simulink model "demapper_simulink"  (R2023a)
settings: Solver=VariableStepAuto  StartTime=0.0  StopTime=976  RelTol=1e-3
libraries: simulink x6
settings Model: Creator=usradmin  LastModifiedBy=usradmin

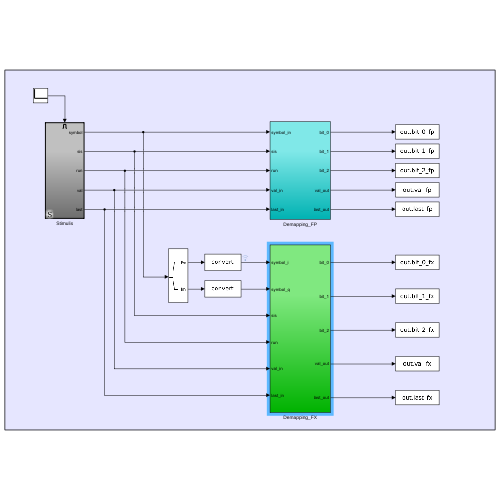
[thumbnail: Simulink's stored preview of the top-level diagram]
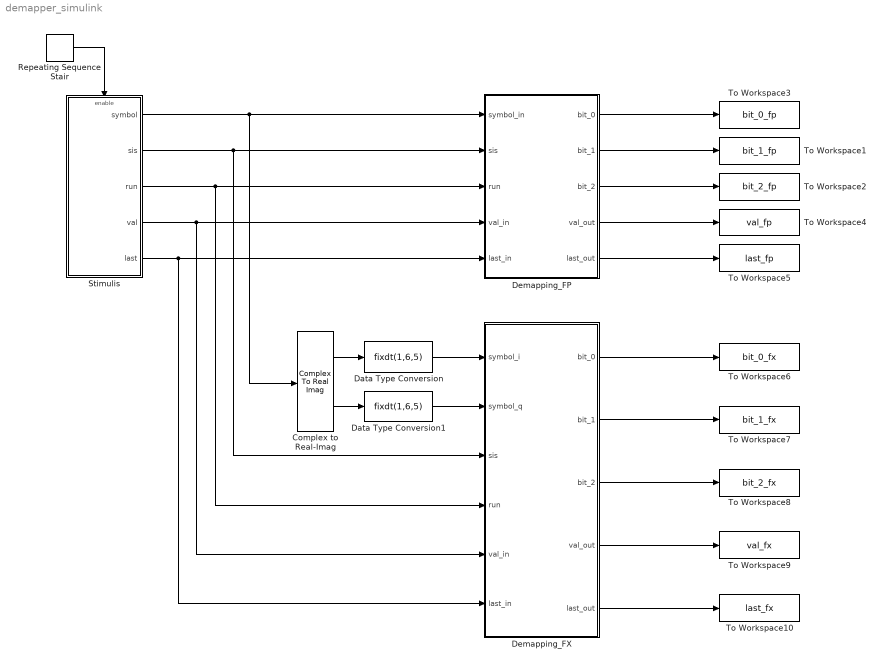
== system demapper_simulink ==
  Complex to Real-Imag : ComplexToRealImag
  Data Type Conversion : DataTypeConversion  OutDataTypeStr=fixdt(1,6,5)  SaturateOnIntegerOverflow=off  RndMeth=Floor
  Data Type Conversion1 : DataTypeConversion  OutDataTypeStr=fixdt(1,6,5)  SaturateOnIntegerOverflow=off  RndMeth=Floor
  Demapping_FP : Subsystem
  Demapping_FX : Subsystem
  Repeating Sequence Stair : simulink/Sources/Repeating Sequence Stair  OutValues=[1].'  tsamp=1  OutMin=[]  OutMax=[]  OutDataTypeStr=double  OutputDataTypeScalingMode=double  OutDataType=fixdt(0,8)  ConRadixGroup=Best Precision: Vector-wise  OutScaling=2^-12
  Stimulis : Subsystem
  To Workspace1 : ToWorkspace  VariableName=bit_1_fp  SaveFormat=Timeseries  SampleTime=-1
  To Workspace10 : ToWorkspace  VariableName=last_fx  SaveFormat=Timeseries  SampleTime=-1
  To Workspace2 : ToWorkspace  VariableName=bit_2_fp  SaveFormat=Timeseries  SampleTime=-1
  To Workspace3 : ToWorkspace  VariableName=bit_0_fp  SaveFormat=Timeseries  SampleTime=-1
  To Workspace4 : ToWorkspace  VariableName=val_fp  SaveFormat=Timeseries  SampleTime=-1
  To Workspace5 : ToWorkspace  VariableName=last_fp  SaveFormat=Timeseries  SampleTime=-1
  To Workspace6 : ToWorkspace  VariableName=bit_0_fx  SaveFormat=Timeseries  SampleTime=-1
  To Workspace7 : ToWorkspace  VariableName=bit_1_fx  SaveFormat=Timeseries  SampleTime=-1
  To Workspace8 : ToWorkspace  VariableName=bit_2_fx  SaveFormat=Timeseries  SampleTime=-1
  To Workspace9 : ToWorkspace  VariableName=val_fx  SaveFormat=Timeseries  SampleTime=-1
  wires:
  Repeating Sequence Stair/1 -> Stimulis/Enable
  Data Type Conversion/1 -> Demapping_FX/1(symbol_i)
  Data Type Conversion1/1 -> Demapping_FX/2(symbol_q)
  Stimulis/2(sis) -> Demapping_FX/3(sis), Demapping_FP/2(sis)
  Complex to Real-Imag/1 -> Data Type Conversion/1
  Complex to Real-Imag/2 -> Data Type Conversion1/1
  Stimulis/1(symbol) -> Complex to Real-Imag/1, Demapping_FP/1(symbol_in)
  Stimulis/3(run) -> Demapping_FX/4(run), Demapping_FP/3(run)
  Stimulis/4(val) -> Demapping_FX/5(val_in), Demapping_FP/4(val_in)
  Stimulis/5(last) -> Demapping_FX/6(last_in), Demapping_FP/5(last_in)
  Demapping_FP/1(bit_0) -> To Workspace3/1
  Demapping_FP/2(bit_1) -> To Workspace1/1
  Demapping_FP/3(bit_2) -> To Workspace2/1
  Demapping_FP/4(val_out) -> To Workspace4/1
  Demapping_FP/5(last_out) -> To Workspace5/1
  Demapping_FX/1(bit_0) -> To Workspace6/1
  Demapping_FX/2(bit_1) -> To Workspace7/1
  Demapping_FX/3(bit_2) -> To Workspace8/1
  Demapping_FX/4(val_out) -> To Workspace9/1
  Demapping_FX/5(last_out) -> To Workspace10/1

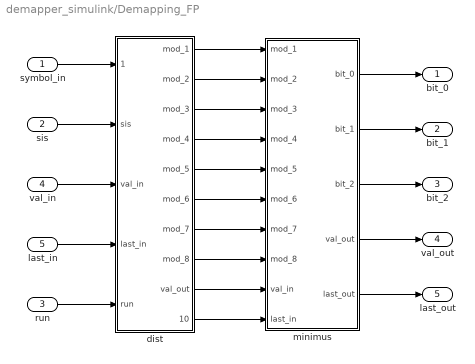
== system demapper_simulink/Demapping_FP ==
  symbol_in : Inport
  sis : Inport  Port=2
  run : Inport  Port=3
  val_in : Inport  Port=4
  last_in : Inport  Port=5
  dist : Subsystem
  minimus : Subsystem
  bit_0 : Outport
  bit_1 : Outport  Port=2
  bit_2 : Outport  Port=3
  val_out : Outport  Port=4
  last_out : Outport  Port=5
  wires:
  minimus/5(last_out) -> last_out/1
  minimus/4(val_out) -> val_out/1
  dist/10(last_out) -> minimus/10(last_in)
  dist/9(val_out) -> minimus/9(val_in)
  run/1 -> dist/5(run)
  last_in/1 -> dist/4(last_in)
  val_in/1 -> dist/3(val_in)
  dist/8(mod_8) -> minimus/8(mod_8)
  dist/7(mod_7) -> minimus/7(mod_7)
  dist/6(mod_6) -> minimus/6(mod_6)
  dist/5(mod_5) -> minimus/5(mod_5)
  dist/4(mod_4) -> minimus/4(mod_4)
  dist/3(mod_3) -> minimus/3(mod_3)
  dist/2(mod_2) -> minimus/2(mod_2)
  minimus/2(bit_1) -> bit_1/1
  minimus/1(bit_0) -> bit_0/1
  dist/1(mod_1) -> minimus/1(mod_1)
  sis/1 -> dist/2(sis)
  minimus/3(bit_2) -> bit_2/1
  symbol_in/1 -> dist/1(symbo_in)

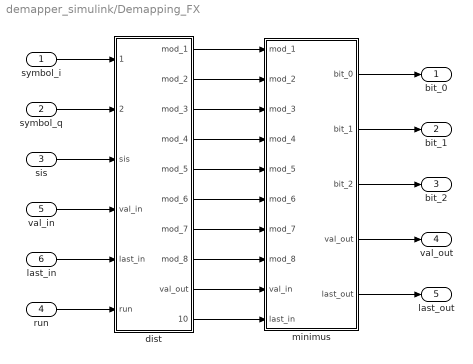
== system demapper_simulink/Demapping_FX ==
  symbol_i : Inport
  symbol_q : Inport  Port=2
  sis : Inport  Port=3
  run : Inport  Port=4
  val_in : Inport  Port=5
  last_in : Inport  Port=6
  dist : Subsystem
  minimus : Subsystem
  bit_0 : Outport
  bit_1 : Outport  Port=2
  bit_2 : Outport  Port=3
  val_out : Outport  Port=4
  last_out : Outport  Port=5
  wires:
  symbol_i/1 -> dist/1(symbol_i)
  symbol_q/1 -> dist/2(symbol_q)
  minimus/3(bit_2) -> bit_2/1
  sis/1 -> dist/3(sis)
  dist/1(mod_1) -> minimus/1(mod_1)
  minimus/1(bit_0) -> bit_0/1
  minimus/2(bit_1) -> bit_1/1
  dist/2(mod_2) -> minimus/2(mod_2)
  dist/3(mod_3) -> minimus/3(mod_3)
  dist/4(mod_4) -> minimus/4(mod_4)
  dist/5(mod_5) -> minimus/5(mod_5)
  dist/6(mod_6) -> minimus/6(mod_6)
  dist/7(mod_7) -> minimus/7(mod_7)
  dist/8(mod_8) -> minimus/8(mod_8)
  val_in/1 -> dist/4(val_in)
  last_in/1 -> dist/5(last_in)
  run/1 -> dist/6(run)
  dist/9(val_out) -> minimus/9(val_in)
  dist/10(last_out) -> minimus/10(last_in)
  minimus/4(val_out) -> val_out/1
  minimus/5(last_out) -> last_out/1

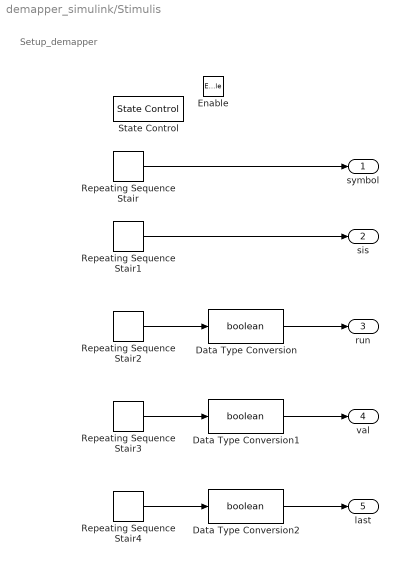
== system demapper_simulink/Stimulis ==
  note: Setup_demapper
  Enable : EnablePort
  Data Type Conversion : DataTypeConversion  OutDataTypeStr=boolean  SaturateOnIntegerOverflow=off  RndMeth=Floor
  Data Type Conversion1 : DataTypeConversion  OutDataTypeStr=boolean  SaturateOnIntegerOverflow=off  RndMeth=Floor
  Data Type Conversion2 : DataTypeConversion  OutDataTypeStr=boolean  SaturateOnIntegerOverflow=off  RndMeth=Floor
  Repeating Sequence Stair : simulink/Sources/Repeating Sequence Stair  OutValues=symbol_cc  tsamp=1  OutMin=[]  OutMax=[]  OutDataTypeStr=double  OutputDataTypeScalingMode=double  OutDataType=fixdt(0,8)  ConRadixGroup=Best Precision: Vector-wise  OutScaling=2^-12
  Repeating Sequence Stair1 : simulink/Sources/Repeating Sequence Stair  OutValues=sis  tsamp=1  OutMin=[]  OutMax=[]  OutDataTypeStr=double  OutputDataTypeScalingMode=double  OutDataType=fixdt(0,8)  ConRadixGroup=Best Precision: Vector-wise  OutScaling=2^-12
  Repeating Sequence Stair2 : simulink/Sources/Repeating Sequence Stair  OutValues=run  tsamp=1  OutMin=[]  OutMax=[]  OutDataTypeStr=double  OutputDataTypeScalingMode=double  OutDataType=fixdt(0,8)  ConRadixGroup=Best Precision: Vector-wise  OutScaling=2^-12
  Repeating Sequence Stair3 : simulink/Sources/Repeating Sequence Stair  OutValues=val  tsamp=1  OutMin=[]  OutMax=[]  OutDataTypeStr=double  OutputDataTypeScalingMode=double  OutDataType=fixdt(0,8)  ConRadixGroup=Best Precision: Vector-wise  OutScaling=2^-12
  Repeating Sequence Stair4 : simulink/Sources/Repeating Sequence Stair  OutValues=last  tsamp=1  OutMin=[]  OutMax=[]  OutDataTypeStr=double  OutputDataTypeScalingMode=double  OutDataType=fixdt(0,8)  ConRadixGroup=Best Precision: Vector-wise  OutScaling=2^-12
  State Control : StateControl  StateControl=Synchronous
  symbol : Outport  VectorParamsAs1DForOutWhenUnconnected=off
  sis : Outport  Port=2  VectorParamsAs1DForOutWhenUnconnected=off
  run : Outport  Port=3  VectorParamsAs1DForOutWhenUnconnected=off
  val : Outport  Port=4  VectorParamsAs1DForOutWhenUnconnected=off
  last : Outport  Port=5  VectorParamsAs1DForOutWhenUnconnected=off
  wires:
  Repeating Sequence Stair/1 -> symbol/1
  Repeating Sequence Stair1/1 -> sis/1
  Repeating Sequence Stair2/1 -> Data Type Conversion/1
  Repeating Sequence Stair3/1 -> Data Type Conversion1/1
  Repeating Sequence Stair4/1 -> Data Type Conversion2/1
  Data Type Conversion/1 -> run/1
  Data Type Conversion1/1 -> val/1
  Data Type Conversion2/1 -> last/1

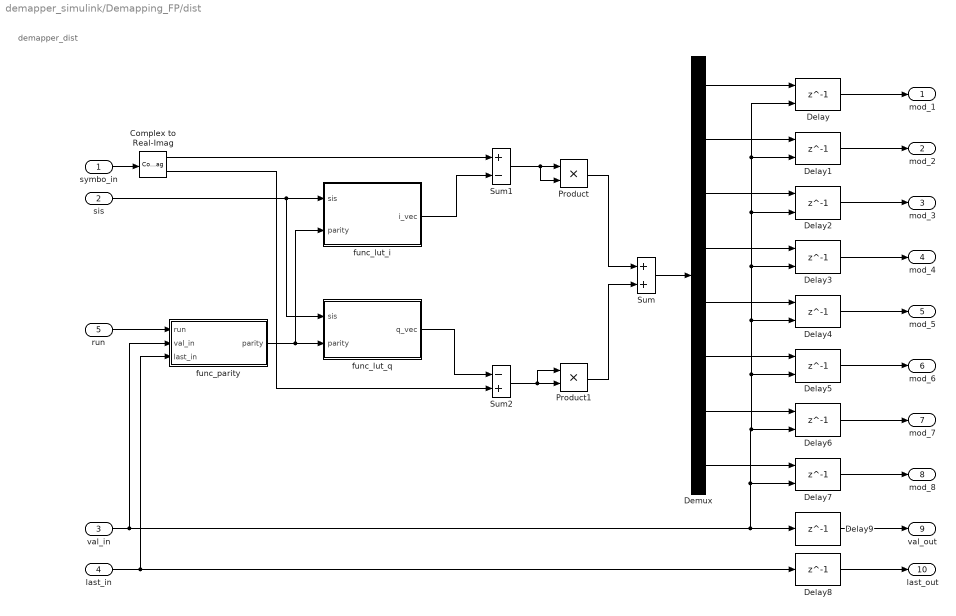
== system demapper_simulink/Demapping_FP/dist ==
  note: demapper_dist
  symbo_in : Inport
  sis : Inport  Port=2
  val_in : Inport  Port=3
  last_in : Inport  Port=4
  run : Inport  Port=5
  Complex to Real-Imag : ComplexToRealImag
  Delay{,1..7} (8 alike) : Delay  DelayLength=1  InitialCondition=0  ShowEnablePort=on
      settings: InputPortMap=u0,e6
  Delay8 : Delay  DelayLength=1  InitialCondition=0
  Delay9 : Delay  DelayLength=1  InitialCondition=0
  Demux : Demux  Outputs=8
  Product : Product
  Product1 : Product
  Sum : Sum
  Sum1 : Sum  Inputs=+-
  Sum2 : Sum  Inputs=-+
  func_lut_i : MATLAB Function  TreatAsAtomicUnit=on
  func_lut_q : MATLAB Function  TreatAsAtomicUnit=on
  func_parity : MATLAB Function  TreatAsAtomicUnit=on
  mod_1 : Outport
  mod_2 : Outport  Port=2
  mod_3 : Outport  Port=3
  mod_4 : Outport  Port=4
  mod_5 : Outport  Port=5
  mod_6 : Outport  Port=6
  mod_7 : Outport  Port=7
  mod_8 : Outport  Port=8
  val_out : Outport  Port=9
  last_out : Outport  Port=10
  wires:
  run/1 -> func_parity/1(run)
  Delay9/1 -> val_out/1
  Delay8/1 -> last_out/1
  last_in/1 -> func_parity/3(last_in), Delay8/1
  Delay7/1 -> mod_8/1
  Delay6/1 -> mod_7/1
  Delay5/1 -> mod_6/1
  Delay4/1 -> mod_5/1
  Delay3/1 -> mod_4/1
  Delay2/1 -> mod_3/1
  Delay1/1 -> mod_2/1
  val_in/1 -> func_parity/2(val_in), Delay9/1, Delay7/2, Delay6/2, Delay5/2, Delay4/2, Delay3/2, Delay2/2, Delay1/2, Delay/2
  Demux/8 -> Delay7/1
  Demux/7 -> Delay6/1
  Demux/6 -> Delay5/1
  Demux/5 -> Delay4/1
  Demux/4 -> Delay3/1
  Demux/3 -> Delay2/1
  Demux/2 -> Delay1/1
  Delay/1 -> mod_1/1
  Demux/1 -> Delay/1
  Sum/1 -> Demux/1
  func_parity/1(parity) -> func_lut_q/2(parity), func_lut_i/2(parity)
  func_lut_q/1(q_vec) -> Sum2/1
  func_lut_i/1(i_vec) -> Sum1/2
  Complex to Real-Imag/2 -> Sum2/2
  Product1/1 -> Sum/2
  Product/1 -> Sum/1
  Sum2/1 -> Product1/2, Product1/1
  sis/1 -> func_lut_i/1(sis), func_lut_q/1(sis)
  Sum1/1 -> Product/1, Product/2
  Complex to Real-Imag/1 -> Sum1/1
  symbo_in/1 -> Complex to Real-Imag/1

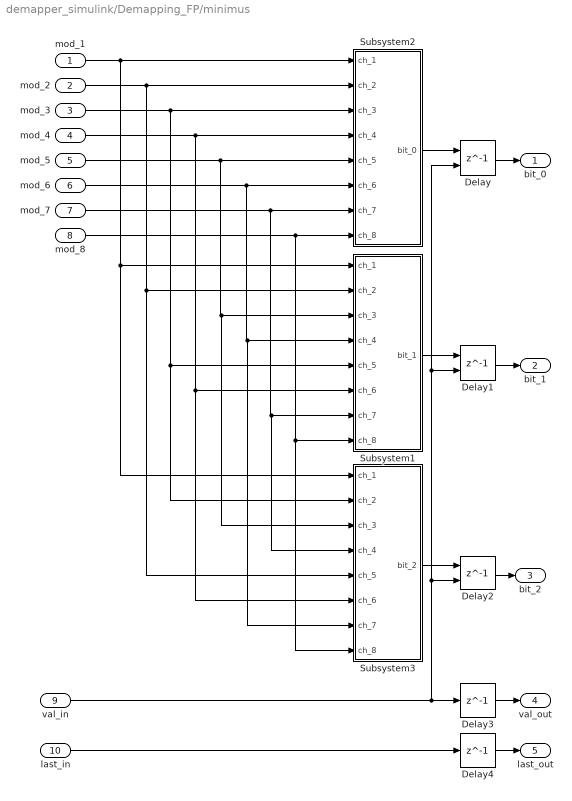
== system demapper_simulink/Demapping_FP/minimus ==
  mod_1 : Inport
  mod_2 : Inport  Port=2
  mod_3 : Inport  Port=3
  mod_4 : Inport  Port=4
  mod_5 : Inport  Port=5
  mod_6 : Inport  Port=6
  mod_7 : Inport  Port=7
  mod_8 : Inport  Port=8
  val_in : Inport  Port=9
  last_in : Inport  Port=10
  Delay : Delay  DelayLength=1  InitialCondition=0  ShowEnablePort=on
      settings: InputPortMap=u0,e6
  Delay1 : Delay  DelayLength=1  InitialCondition=0  ShowEnablePort=on
      settings: InputPortMap=u0,e6
  Delay2 : Delay  DelayLength=1  InitialCondition=0  ShowEnablePort=on
      settings: InputPortMap=u0,e6
  Delay3 : Delay  DelayLength=1  InitialCondition=0
  Delay4 : Delay  DelayLength=1  InitialCondition=0
  Subsystem1 : Subsystem
  Subsystem2 : Subsystem
  Subsystem3 : Subsystem
  bit_0 : Outport  VectorParamsAs1DForOutWhenUnconnected=off
  bit_1 : Outport  Port=2  VectorParamsAs1DForOutWhenUnconnected=off
  bit_2 : Outport  Port=3  VectorParamsAs1DForOutWhenUnconnected=off
  val_out : Outport  Port=4  VectorParamsAs1DForOutWhenUnconnected=off
  last_out : Outport  Port=5  VectorParamsAs1DForOutWhenUnconnected=off
  wires:
  Delay4/1 -> last_out/1
  last_in/1 -> Delay4/1
  Delay3/1 -> val_out/1
  val_in/1 -> Delay3/1, Delay2/2, Delay1/2, Delay/2
  Delay2/1 -> bit_2/1
  Delay1/1 -> bit_1/1
  Delay/1 -> bit_0/1
  mod_7/1 -> Subsystem1/7(ch_7), Subsystem3/4(ch_4), Subsystem2/7(ch_7)
  mod_2/1 -> Subsystem2/2(ch_2), Subsystem1/2(ch_2), Subsystem3/5(ch_5)
  mod_6/1 -> Subsystem3/7(ch_7), Subsystem1/4(ch_4), Subsystem2/6(ch_6)
  mod_1/1 -> Subsystem2/1(ch_1), Subsystem1/1(ch_1), Subsystem3/1(ch_1)
  mod_4/1 -> Subsystem1/6(ch_6), Subsystem3/6(ch_6), Subsystem2/4(ch_4)
  mod_8/1 -> Subsystem3/8(ch_8), Subsystem1/8(ch_8), Subsystem2/8(ch_8)
  Subsystem2/1(bit_0) -> Delay/1
  Subsystem3/1(bit_2) -> Delay2/1
  Subsystem1/1(bit_1) -> Delay1/1
  mod_3/1 -> Subsystem2/3(ch_3), Subsystem3/2(ch_2), Subsystem1/5(ch_5)
  mod_5/1 -> Subsystem2/5(ch_5), Subsystem1/3(ch_3), Subsystem3/3(ch_3)

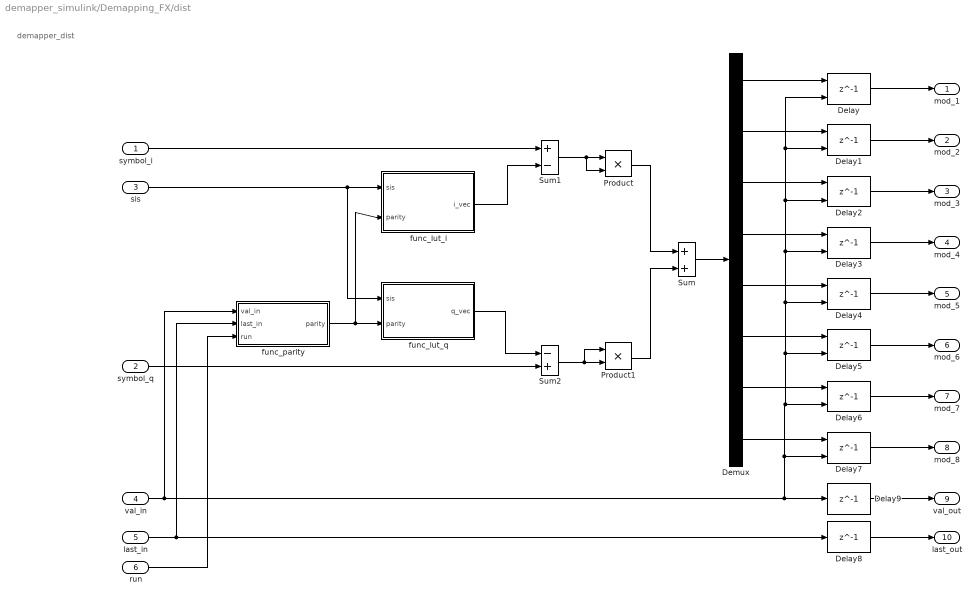
== system demapper_simulink/Demapping_FX/dist ==
  note: demapper_dist
  symbol_i : Inport
  symbol_q : Inport  Port=2
  sis : Inport  Port=3
  val_in : Inport  Port=4
  last_in : Inport  Port=5
  run : Inport  Port=6
  Delay{,1..7} (8 alike) : Delay  DelayLength=1  InitialCondition=0  ShowEnablePort=on
      settings: InputPortMap=u0,e6
  Delay8 : Delay  DelayLength=1  InitialCondition=0
  Delay9 : Delay  DelayLength=1  InitialCondition=0
  Demux : Demux  Outputs=8
  Product : Product
  Product1 : Product
  Sum : Sum
  Sum1 : Sum  Inputs=+-
  Sum2 : Sum  Inputs=-+
  func_lut_i : MATLAB Function  TreatAsAtomicUnit=on
  func_lut_q : MATLAB Function  TreatAsAtomicUnit=on
  func_parity : MATLAB Function  TreatAsAtomicUnit=on
  mod_1 : Outport
  mod_2 : Outport  Port=2
  mod_3 : Outport  Port=3
  mod_4 : Outport  Port=4
  mod_5 : Outport  Port=5
  mod_6 : Outport  Port=6
  mod_7 : Outport  Port=7
  mod_8 : Outport  Port=8
  val_out : Outport  Port=9
  last_out : Outport  Port=10
  wires:
  Sum1/1 -> Product/2, Product/1
  sis/1 -> func_lut_q/1(sis), func_lut_i/1(sis)
  Sum2/1 -> Product1/1, Product1/2
  symbol_i/1 -> Sum1/1
  Product/1 -> Sum/1
  Product1/1 -> Sum/2
  symbol_q/1 -> Sum2/2
  func_lut_i/1(i_vec) -> Sum1/2
  func_lut_q/1(q_vec) -> Sum2/1
  func_parity/1(parity) -> func_lut_i/2(parity), func_lut_q/2(parity)
  Sum/1 -> Demux/1
  Demux/1 -> Delay/1
  Delay/1 -> mod_1/1
  Demux/2 -> Delay1/1
  Demux/3 -> Delay2/1
  Demux/4 -> Delay3/1
  Demux/5 -> Delay4/1
  Demux/6 -> Delay5/1
  Demux/7 -> Delay6/1
  Demux/8 -> Delay7/1
  val_in/1 -> Delay/2, Delay1/2, Delay2/2, Delay3/2, Delay4/2, Delay5/2, Delay6/2, Delay7/2, Delay9/1, func_parity/1(val_in)
  Delay1/1 -> mod_2/1
  Delay2/1 -> mod_3/1
  Delay3/1 -> mod_4/1
  Delay4/1 -> mod_5/1
  Delay5/1 -> mod_6/1
  Delay6/1 -> mod_7/1
  Delay7/1 -> mod_8/1
  last_in/1 -> Delay8/1, func_parity/2(last_in)
  Delay8/1 -> last_out/1
  Delay9/1 -> val_out/1
  run/1 -> func_parity/3(run)

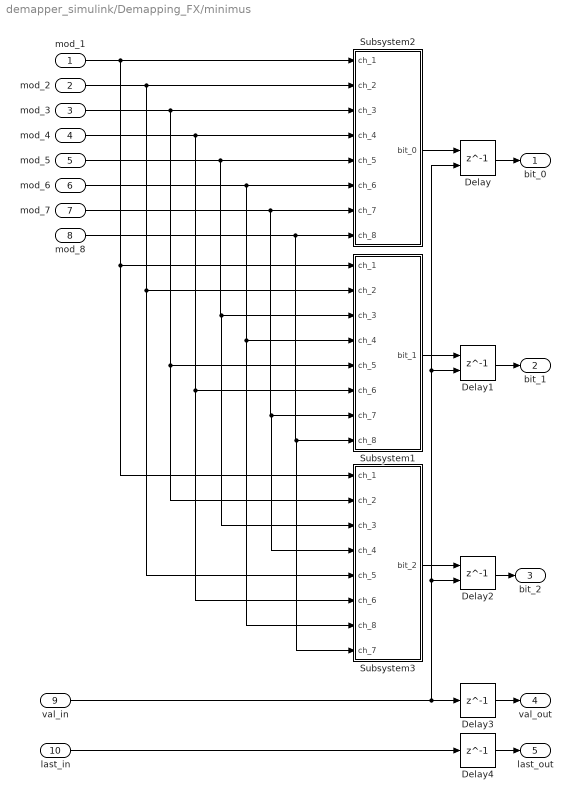
== system demapper_simulink/Demapping_FX/minimus ==
  mod_1 : Inport
  mod_2 : Inport  Port=2
  mod_3 : Inport  Port=3
  mod_4 : Inport  Port=4
  mod_5 : Inport  Port=5
  mod_6 : Inport  Port=6
  mod_7 : Inport  Port=7
  mod_8 : Inport  Port=8
  val_in : Inport  Port=9
  last_in : Inport  Port=10
  Delay : Delay  DelayLength=1  InitialCondition=0  ShowEnablePort=on
      settings: InputPortMap=u0,e6
  Delay1 : Delay  DelayLength=1  InitialCondition=0  ShowEnablePort=on
      settings: InputPortMap=u0,e6
  Delay2 : Delay  DelayLength=1  InitialCondition=0  ShowEnablePort=on
      settings: InputPortMap=u0,e6
  Delay3 : Delay  DelayLength=1  InitialCondition=0
  Delay4 : Delay  DelayLength=1  InitialCondition=0
  Subsystem1 : Subsystem
  Subsystem2 : Subsystem
  Subsystem3 : Subsystem
  bit_0 : Outport  VectorParamsAs1DForOutWhenUnconnected=off
  bit_1 : Outport  Port=2  VectorParamsAs1DForOutWhenUnconnected=off
  bit_2 : Outport  Port=3  VectorParamsAs1DForOutWhenUnconnected=off
  val_out : Outport  Port=4  VectorParamsAs1DForOutWhenUnconnected=off
  last_out : Outport  Port=5  VectorParamsAs1DForOutWhenUnconnected=off
  wires:
  mod_5/1 -> Subsystem3/3(ch_3), Subsystem1/3(ch_3), Subsystem2/5(ch_5)
  mod_3/1 -> Subsystem1/5(ch_5), Subsystem3/2(ch_2), Subsystem2/3(ch_3)
  Subsystem1/1(bit_1) -> Delay1/1
  Subsystem3/1(bit_2) -> Delay2/1
  Subsystem2/1(bit_0) -> Delay/1
  mod_8/1 -> Subsystem2/8(ch_8), Subsystem3/8(ch_7), Subsystem1/8(ch_8)
  mod_4/1 -> Subsystem2/4(ch_4), Subsystem3/6(ch_6), Subsystem1/6(ch_6)
  mod_1/1 -> Subsystem3/1(ch_1), Subsystem1/1(ch_1), Subsystem2/1(ch_1)
  mod_6/1 -> Subsystem2/6(ch_6), Subsystem3/7(ch_8), Subsystem1/4(ch_4)
  mod_2/1 -> Subsystem3/5(ch_5), Subsystem1/2(ch_2), Subsystem2/2(ch_2)
  mod_7/1 -> Subsystem2/7(ch_7), Subsystem3/4(ch_4), Subsystem1/7(ch_7)
  Delay/1 -> bit_0/1
  Delay1/1 -> bit_1/1
  Delay2/1 -> bit_2/1
  val_in/1 -> Delay/2, Delay1/2, Delay2/2, Delay3/1
  Delay3/1 -> val_out/1
  last_in/1 -> Delay4/1
  Delay4/1 -> last_out/1

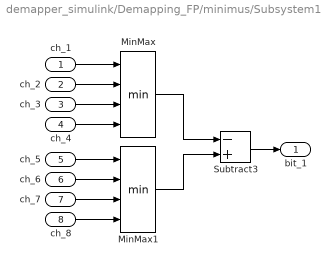
== system demapper_simulink/Demapping_FP/minimus/Subsystem1 ==
  ch_1 : Inport
  ch_2 : Inport  Port=2
  ch_3 : Inport  Port=3
  ch_4 : Inport  Port=4
  ch_5 : Inport  Port=5
  ch_6 : Inport  Port=6
  ch_7 : Inport  Port=7
  ch_8 : Inport  Port=8
  MinMax : MinMax  Inputs=4
  MinMax1 : MinMax  Inputs=4
  Subtract3 : Sum  Inputs=-+
  bit_1 : Outport
  wires:
  ch_7/1 -> MinMax1/3
  ch_8/1 -> MinMax1/4
  Subtract3/1 -> bit_1/1
  ch_5/1 -> MinMax1/1
  MinMax1/1 -> Subtract3/2
  ch_6/1 -> MinMax1/2
  MinMax/1 -> Subtract3/1
  ch_1/1 -> MinMax/1
  ch_3/1 -> MinMax/3
  ch_2/1 -> MinMax/2
  ch_4/1 -> MinMax/4

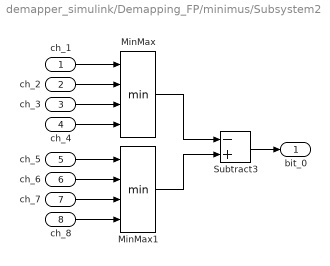
== system demapper_simulink/Demapping_FP/minimus/Subsystem2 ==
  ch_1 : Inport
  ch_2 : Inport  Port=2
  ch_3 : Inport  Port=3
  ch_4 : Inport  Port=4
  ch_5 : Inport  Port=5
  ch_6 : Inport  Port=6
  ch_7 : Inport  Port=7
  ch_8 : Inport  Port=8
  MinMax : MinMax  Inputs=4
  MinMax1 : MinMax  Inputs=4
  Subtract3 : Sum  Inputs=-+
  bit_0 : Outport
  wires:
  ch_4/1 -> MinMax/4
  ch_2/1 -> MinMax/2
  ch_3/1 -> MinMax/3
  ch_1/1 -> MinMax/1
  MinMax/1 -> Subtract3/1
  ch_6/1 -> MinMax1/2
  MinMax1/1 -> Subtract3/2
  ch_5/1 -> MinMax1/1
  Subtract3/1 -> bit_0/1
  ch_8/1 -> MinMax1/4
  ch_7/1 -> MinMax1/3

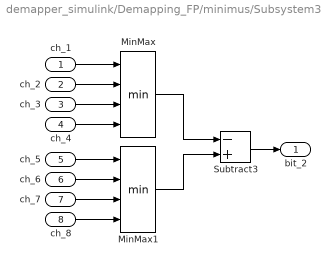
== system demapper_simulink/Demapping_FP/minimus/Subsystem3 ==
  ch_1 : Inport
  ch_2 : Inport  Port=2
  ch_3 : Inport  Port=3
  ch_4 : Inport  Port=4
  ch_5 : Inport  Port=5
  ch_6 : Inport  Port=6
  ch_7 : Inport  Port=7
  ch_8 : Inport  Port=8
  MinMax : MinMax  Inputs=4
  MinMax1 : MinMax  Inputs=4
  Subtract3 : Sum  Inputs=-+
  bit_2 : Outport
  wires:
  ch_4/1 -> MinMax/4
  ch_2/1 -> MinMax/2
  ch_3/1 -> MinMax/3
  ch_1/1 -> MinMax/1
  MinMax/1 -> Subtract3/1
  ch_6/1 -> MinMax1/2
  MinMax1/1 -> Subtract3/2
  ch_5/1 -> MinMax1/1
  Subtract3/1 -> bit_2/1
  ch_8/1 -> MinMax1/4
  ch_7/1 -> MinMax1/3

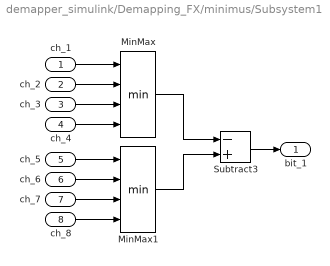
== system demapper_simulink/Demapping_FX/minimus/Subsystem1 ==
  ch_1 : Inport
  ch_2 : Inport  Port=2
  ch_3 : Inport  Port=3
  ch_4 : Inport  Port=4
  ch_5 : Inport  Port=5
  ch_6 : Inport  Port=6
  ch_7 : Inport  Port=7
  ch_8 : Inport  Port=8
  MinMax : MinMax  Inputs=4
  MinMax1 : MinMax  Inputs=4
  Subtract3 : Sum  Inputs=-+
  bit_1 : Outport
  wires:
  ch_4/1 -> MinMax/4
  ch_2/1 -> MinMax/2
  ch_3/1 -> MinMax/3
  ch_1/1 -> MinMax/1
  MinMax/1 -> Subtract3/1
  ch_6/1 -> MinMax1/2
  MinMax1/1 -> Subtract3/2
  ch_5/1 -> MinMax1/1
  Subtract3/1 -> bit_1/1
  ch_8/1 -> MinMax1/4
  ch_7/1 -> MinMax1/3

== system demapper_simulink/Demapping_FX/minimus/Subsystem2 ==
  ch_1 : Inport
  ch_2 : Inport  Port=2
  ch_3 : Inport  Port=3
  ch_4 : Inport  Port=4
  ch_5 : Inport  Port=5
  ch_6 : Inport  Port=6
  ch_7 : Inport  Port=7
  ch_8 : Inport  Port=8
  MinMax : MinMax  Inputs=4
  MinMax1 : MinMax  Inputs=4
  Subtract3 : Sum  Inputs=-+
  bit_0 : Outport
  wires:
  ch_7/1 -> MinMax1/3
  ch_8/1 -> MinMax1/4
  Subtract3/1 -> bit_0/1
  ch_5/1 -> MinMax1/1
  MinMax1/1 -> Subtract3/2
  ch_6/1 -> MinMax1/2
  MinMax/1 -> Subtract3/1
  ch_1/1 -> MinMax/1
  ch_3/1 -> MinMax/3
  ch_2/1 -> MinMax/2
  ch_4/1 -> MinMax/4

== system demapper_simulink/Demapping_FX/minimus/Subsystem3 ==
  ch_1 : Inport
  ch_2 : Inport  Port=2
  ch_3 : Inport  Port=3
  ch_4 : Inport  Port=4
  ch_5 : Inport  Port=5
  ch_6 : Inport  Port=6
  ch_8 : Inport  Port=7
  ch_7 : Inport  Port=8
  MinMax : MinMax  Inputs=4
  MinMax1 : MinMax  Inputs=4
  Subtract3 : Sum  Inputs=-+
  bit_2 : Outport
  wires:
  ch_7/1 -> MinMax1/3
  ch_8/1 -> MinMax1/4
  Subtract3/1 -> bit_2/1
  ch_5/1 -> MinMax1/1
  MinMax1/1 -> Subtract3/2
  ch_6/1 -> MinMax1/2
  MinMax/1 -> Subtract3/1
  ch_1/1 -> MinMax/1
  ch_3/1 -> MinMax/3
  ch_2/1 -> MinMax/2
  ch_4/1 -> MinMax/4

== matlab function demapper_simulink/Demapping_FX/dist/func_lut_q ==
  data: sis input; q_vec output; parity input
function q_vec = func_lut_q(sis, parity)
%#codegen

    if (sis == 1 && parity == 0)
        Q_1 =  0;
        Q_2 =  3;
        Q_3 =  3;
        Q_4 =  3;
        Q_5 =  3;
        Q_6 =  3;
        Q_7 =  0;
        Q_8 =  3;
    
    elseif (sis == 1 && parity == 1)
        Q_1 = 0;
        Q_2 =  3;
        Q_3 =  3;
        Q_4 =  1;
        Q_5 =  3;
        Q_6 = -1;
        Q_7 =  0;
        Q_8 =  3;
    
    elseif (sis == 2 && parity == 0)
        Q_1 =  0; 
        Q_2 =  0.7071;
        Q_3 =  0.7071;
        Q_4 =  1;
        Q_5 = -0.7071;
        Q_6 = -1;
        Q_7 =  0;
        Q_8 = -0.7071;
    
    elseif (sis == 2 && parity == 1)
        Q_1 = 1;
        Q_2 = 3;
        Q_3 = 3;
        Q_4 = 3;
        Q_5 = 3;
        Q_6 = 3;
        Q_7 = -1;
        Q_8 = 3;
    
    elseif (sis == 3 && parity == 0)
        Q_1 =  0.7071; 
        Q_2 =  3;
        Q_3 =  3;
        Q_4 =  0.7071;
        Q_5 =  3;
        Q_6 = -0.7071;
        Q_7 = -0.7071;
        Q_8 =  3;
    
    else
        Q_1 =  0.3827;
        Q_2 =  0.9239;
        Q_3 =  0.3827;
        Q_4 =  0.9239;
        Q_5 = -0.3827;
        Q_6 = -0.9238;
        Q_7 = -0.3827;
        Q_8 = -0.9239;
    end 
    q_vec = [Q_1; Q_2; Q_3; Q_4; Q_5; Q_6; Q_7; Q_8];

end

== matlab function demapper_simulink/Demapping_FX/dist/func_lut_i ==
  data: sis input; i_vec output; parity input
function i_vec = func_lut_i(sis, parity)
%#codegen

    if (sis == 1 && parity == 0)
        I_1 = 1;
        I_2 = 3;
        I_3 = 3;
        I_4 = 3;
        I_5 = 3;
        I_6 = 3;
        I_7 = -1;
        I_8 = 3;
    
    elseif (sis == 1 && parity == 1)
        I_1 = 1;
        I_2 = 3;
        I_3 = 3;
        I_4 = 0;
        I_5 = 3;
        I_6 = 0;
        I_7 = -1;
        I_8 = 3;
    
    elseif (sis == 2 && parity == 0)
        I_1 = 1; 
        I_2 = 0.7071;
        I_3 = -0.7071;
        I_4 = 0;
        I_5 = 0.7071;
        I_6 = 0;
        I_7 = -1;
        I_8 = -0.7071;
    
    elseif (sis == 2 && parity == 1)
        I_1 = 0;
        I_2 = 3;
        I_3 = 3;
        I_4 = 3;
        I_5 = 3;
        I_6 = 3;
        I_7 = 0;
        I_8 = 3;
    
    elseif (sis == 3 && parity == 0)
        I_1 = 0.7071; 
        I_2 = 3;
        I_3 = 3;
        I_4 = -0.7071;
        I_5 = 3;
        I_6 = 0.7071;
        I_7 = -0.7071;
        I_8 = 3;
    
    else
        I_1 = 0.9239;
        I_2 = 0.3827;
        I_3 = -0.9239;
        I_4 = -0.3827;
        I_5 = 0.9239;
        I_6 = 0.3827;
        I_7 = -0.9239;
        I_8 = -0.3827;
    end 
    i_vec = [I_1; I_2; I_3; I_4; I_5; I_6; I_7; I_8];
end

== matlab function demapper_simulink/Demapping_FX/dist/func_parity ==
  data: val_in input; parity output; last_in input; run input
function parity = func_parity(val_in, last_in, run)
% -------------------------------------------------------------------------
% Function valid
% -------------------------------------------------------------------------
    % persistent variable for the state
    persistent count;
    if isempty(count)
        count = uint16(0);
    end

    persistent parity_int;
    if isempty(parity_int)
        parity_int = false;
    end

    % counting up
    if (not(run))
        count = uint16(0);
    elseif (val_in)
        count = count + uint16(1);
        % limit
        if (last_in || count > uint16(156))
            count = uint16(0);
        end
    end

    if (val_in && count > uint16(156))
        parity_int = false;
    elseif (val_in)
        parity_int = not(parity_int);
    end 

    parity = parity_int;
end

== matlab function demapper_simulink/Demapping_FP/dist/func_lut_i ==
  data: sis input; i_vec output; parity input
function i_vec = func_lut_i(sis, parity)
%#codegen

    if (sis == 1 && parity == 0)
        I_1 = 1;
        I_2 = 3;
        I_3 = 3;
        I_4 = 3;
        I_5 = 3;
        I_6 = 3;
        I_7 = -1;
        I_8 = 3;
    
    elseif (sis == 1 && parity == 1)
        I_1 = 1;
        I_2 = 3;
        I_3 = 3;
        I_4 = 0;
        I_5 = 3;
        I_6 = 0;
        I_7 = -1;
        I_8 = 3;
    
    elseif (sis == 2 && parity == 0)
        I_1 = 1; 
        I_2 = 0.7071;
        I_3 = -0.7071;
        I_4 = 0;
        I_5 = 0.7071;
        I_6 = 0;
        I_7 = -1;
        I_8 = -0.7071;
    
    elseif (sis == 2 && parity == 1)
        I_1 = 0;
        I_2 = 3;
        I_3 = 3;
        I_4 = 3;
        I_5 = 3;
        I_6 = 3;
        I_7 = 0;
        I_8 = 3;
    
    elseif (sis == 3 && parity == 0)
        I_1 = 0.7071; 
        I_2 = 3;
        I_3 = 3;
        I_4 = -0.7071;
        I_5 = 3;
        I_6 = 0.7071;
        I_7 = -0.7071;
        I_8 = 3;
    
    else
        I_1 = 0.9239;
        I_2 = 0.3827;
        I_3 = -0.9239;
        I_4 = -0.3827;
        I_5 = 0.9239;
        I_6 = 0.3827;
        I_7 = -0.9239;
        I_8 = -0.3827;
    end 
    i_vec = [I_1; I_2; I_3; I_4; I_5; I_6; I_7; I_8];
end

== matlab function demapper_simulink/Demapping_FP/dist/func_lut_q ==
  data: sis input; q_vec output; parity input
function q_vec = func_lut_q(sis, parity)
%#codegen

    if (sis == 1 && parity == 0)
        Q_1 =  0;
        Q_2 =  3;
        Q_3 =  3;
        Q_4 =  3;
        Q_5 =  3;
        Q_6 =  3;
        Q_7 =  0;
        Q_8 =  3;
    
    elseif (sis == 1 && parity == 1)
        Q_1 = 0;
        Q_2 =  3;
        Q_3 =  3;
        Q_4 =  1;
        Q_5 =  3;
        Q_6 = -1;
        Q_7 =  0;
        Q_8 =  3;
    
    elseif (sis == 2 && parity == 0)
        Q_1 =  0; 
        Q_2 =  0.7071;
        Q_3 =  0.7071;
        Q_4 =  1;
        Q_5 = -0.7071;
        Q_6 = -1;
        Q_7 =  0;
        Q_8 = -0.7071;
    
    elseif (sis == 2 && parity == 1)
        Q_1 = 1;
        Q_2 = 3;
        Q_3 = 3;
        Q_4 = 3;
        Q_5 = 3;
        Q_6 = 3;
        Q_7 = -1;
        Q_8 = 3;
    
    elseif (sis == 3 && parity == 0)
        Q_1 =  0.7071; 
        Q_2 =  3;
        Q_3 =  3;
        Q_4 =  0.7071;
        Q_5 =  3;
        Q_6 = -0.7071;
        Q_7 = -0.7071;
        Q_8 =  3;
    
    else
        Q_1 =  0.3827;
        Q_2 =  0.9239;
        Q_3 =  0.3827;
        Q_4 =  0.9239;
        Q_5 = -0.3827;
        Q_6 = -0.9238;
        Q_7 = -0.3827;
        Q_8 = -0.9239;
    end 
    q_vec = [Q_1; Q_2; Q_3; Q_4; Q_5; Q_6; Q_7; Q_8];

end

== matlab function demapper_simulink/Demapping_FP/dist/func_parity ==
  data: run input; val_in input; parity output; last_in input
function parity = func_parity(run, val_in, last_in)
% -------------------------------------------------------------------------
% Function valid
% -------------------------------------------------------------------------
    % persistent variable for the state
    persistent count;
    if isempty(count)
        count = uint16(0);
    end

    persistent parity_int;
    if isempty(parity_int)
        parity_int = false;
    end

    % counting up
    if (not(run))
        count = uint16(0);
    elseif (val_in)
        count = count + uint16(1);
        % limit
        if (last_in || count > uint16(156))
            count = uint16(0);
        end
    end

    if (val_in && count > uint16(156))
        parity_int = false;
    elseif (val_in)
        parity_int = not(parity_int);
    end 

    parity = parity_int;
end
